simulink model "FOC_Simulate"  (R2016b)
settings: Solver=ode4  StartTime=0.0  StopTime=15  FixedStep=1e-5  RelTol=1e-3  EnableMultiTasking=on
undefined symbols (not defined in the file): sigbuilder_block
libraries: powerlib_meascontrol x4, powerlib x4, simulink x4
settings Model: ExtModeTrigDuration=8  Creator=tiend  LastModifiedBy=tiend

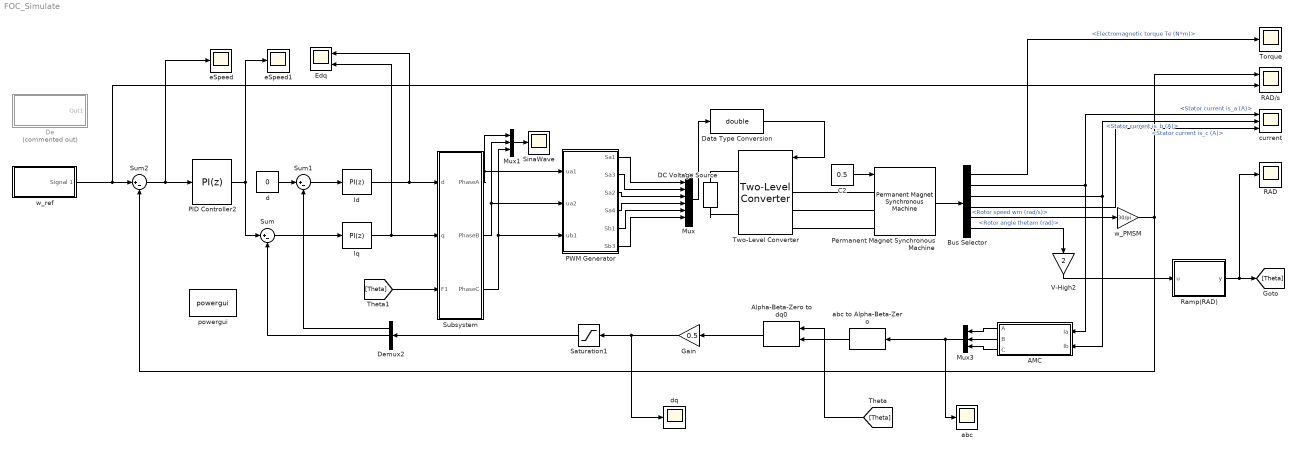
== system FOC_Simulate ==
  AMC : Subsystem
  Alpha-Beta-Zero to dq0 : powerlib_meascontrol/Transformations/Alpha-Beta-Zero to dq0  Alignment=Aligned with phase A axis
  Bus Selector : BusSelector  OutputSignals=Electromagnetic torque Te (N*m),Stator current is_a (A),Stator current is_b (A),Stator current is_c (A),Rotor speed wm (rad/s),Rotor angle thetam (rad)
  C2 : Constant  Value=0.5
  DC Voltage Source : powerlib/Electrical Sources/DC Voltage Source  Amplitude=300  Measurements=Voltage
  Data Type Conversion : DataTypeConversion  OutDataTypeStr=double
  De : Subsystem  Commented=on
  Demux2 : Demux  Outputs=3
  Edq : Scope  NumInputPorts=2
  Gain : Gain  Gain=0.5
  Id : simulink/Continuous/PID Controller  Controller=PI  TimeDomain=Discrete-time  SampleTime=-1  IntegratorMethod=Forward Euler  FilterMethod=Forward Euler  Form=Parallel  UseFilter=on  ControllerParametersSource=internal  P=5  I=0.3  D=0  N=100  InitialConditionSource=internal  InitialConditionForIntegrator=0  InitialConditionForFilter=0  ExternalReset=none  LimitOutput=on  UpperSaturationLimit=1  LowerSaturationLimit=-1  LinearizeAsGain=on  AntiWindupMode=none  Kb=1  TrackingMode=off  Kt=1  PParamMin=[]  PParamMax=[]  IParamMin=[]  IParamMax=[]  DParamMin=[]  DParamMax=[]  NParamMin=[]  NParamMax=[]  KbParamMin=[]  KbParamMax=[]  KtParamMin=[]  KtParamMax=[]  POutMin=[]  POutMax=[]  IOutMin=[]  IOutMax=[]  DOutMin=[]  DOutMax=[]  NOutMin=[]  NOutMax=[]  KbOutMin=[]  KbOutMax=[]  KtOutMin=[]  KtOutMax=[]  IntegratorOutMin=[]  IntegratorOutMax=[]  FilterOutMin=[]  FilterOutMax=[]  SumOutMin=[]  SumOutMax=[]  SumI1OutMin=[]  SumI1OutMax=[]  SumI2OutMin=[]  SumI2OutMax=[]  SumI3OutMin=[]  SumI3OutMax=[]  SumDOutMin=[]  SumDOutMax=[]  SaturationOutMin=[]  SaturationOutMax=[]  IntegratorContinuousStateAttributes=''  IntegratorStateMustResolveToSignalObject=off  IntegratorRTWStateStorageClass=Auto  FilterContinuousStateAttributes=''  FilterStateMustResolveToSignalObject=off  FilterRTWStateStorageClass=Auto  DifferentiatorICPrevScaledInput=0  DifferentiatorOutMin=[]  DifferentiatorOutMax=[]
  Iq : simulink/Continuous/PID Controller  Controller=PI  TimeDomain=Discrete-time  SampleTime=-1  IntegratorMethod=Forward Euler  FilterMethod=Forward Euler  Form=Parallel  UseFilter=on  ControllerParametersSource=internal  P=5  I=0.3  D=0  N=100  InitialConditionSource=internal  InitialConditionForIntegrator=0  InitialConditionForFilter=0  ExternalReset=none  LimitOutput=on  UpperSaturationLimit=1  LowerSaturationLimit=-1  LinearizeAsGain=on  AntiWindupMode=none  Kb=1  TrackingMode=off  Kt=1  PParamMin=[]  PParamMax=[]  IParamMin=[]  IParamMax=[]  DParamMin=[]  DParamMax=[]  NParamMin=[]  NParamMax=[]  KbParamMin=[]  KbParamMax=[]  KtParamMin=[]  KtParamMax=[]  POutMin=[]  POutMax=[]  IOutMin=[]  IOutMax=[]  DOutMin=[]  DOutMax=[]  NOutMin=[]  NOutMax=[]  KbOutMin=[]  KbOutMax=[]  KtOutMin=[]  KtOutMax=[]  IntegratorOutMin=[]  IntegratorOutMax=[]  FilterOutMin=[]  FilterOutMax=[]  SumOutMin=[]  SumOutMax=[]  SumI1OutMin=[]  SumI1OutMax=[]  SumI2OutMin=[]  SumI2OutMax=[]  SumI3OutMin=[]  SumI3OutMax=[]  SumDOutMin=[]  SumDOutMax=[]  SaturationOutMin=[]  SaturationOutMax=[]  IntegratorContinuousStateAttributes=''  IntegratorStateMustResolveToSignalObject=off  IntegratorRTWStateStorageClass=Auto  FilterContinuousStateAttributes=''  FilterStateMustResolveToSignalObject=off  FilterRTWStateStorageClass=Auto  DifferentiatorICPrevScaledInput=0  DifferentiatorOutMin=[]  DifferentiatorOutMax=[]
  Mux : Mux  Inputs=6
  Mux1 : Mux  Inputs=3
  Mux3 : Mux  Inputs=3
  PID Controller2 : simulink/Continuous/PID Controller  Controller=PI  TimeDomain=Discrete-time  SampleTime=-1  IntegratorMethod=Forward Euler  FilterMethod=Forward Euler  Form=Parallel  UseFilter=on  ControllerParametersSource=internal  P=1/900  I=0.005  D=0  N=100  InitialConditionSource=internal  InitialConditionForIntegrator=0  InitialConditionForFilter=0  ExternalReset=none  LimitOutput=off  UpperSaturationLimit=1  LowerSaturationLimit=-1  LinearizeAsGain=on  AntiWindupMode=none  Kb=1  TrackingMode=off  Kt=1  PParamMin=[]  PParamMax=[]  IParamMin=[]  IParamMax=[]  DParamMin=[]  DParamMax=[]  NParamMin=[]  NParamMax=[]  KbParamMin=[]  KbParamMax=[]  KtParamMin=[]  KtParamMax=[]  POutMin=[]  POutMax=[]  IOutMin=[]  IOutMax=[]  DOutMin=[]  DOutMax=[]  NOutMin=[]  NOutMax=[]  KbOutMin=[]  KbOutMax=[]  KtOutMin=[]  KtOutMax=[]  IntegratorOutMin=[]  IntegratorOutMax=[]  FilterOutMin=[]  FilterOutMax=[]  SumOutMin=[]  SumOutMax=[]  SumI1OutMin=[]  SumI1OutMax=[]  SumI2OutMin=[]  SumI2OutMax=[]  SumI3OutMin=[]  SumI3OutMax=[]  SumDOutMin=[]  SumDOutMax=[]  SaturationOutMin=[]  SaturationOutMax=[]  IntegratorContinuousStateAttributes=''  IntegratorStateMustResolveToSignalObject=off  IntegratorRTWStateStorageClass=Auto  FilterContinuousStateAttributes=''  FilterStateMustResolveToSignalObject=off  FilterRTWStateStorageClass=Auto  DifferentiatorICPrevScaledInput=0  DifferentiatorOutMin=[]  DifferentiatorOutMax=[]
  PWM Generator : Subsystem
  Permanent Magnet Synchronous Machine : powerlib/Machines/Permanent Magnet Synchronous Machine  NbPhases=3  FluxDistribution=Sinusoidal  RotorType=Round  MechanicalLoad=Torque Tm  PresetModel="01:  0.8 Nm 300 Vdc 3000 RPM - 0.8 Nm"  ShowDetailedParameters=on  MeasurementBus=off  Resistance=18.7  Inductance=8.5e-3  dqInductances=[0.02547 0.02816]  La=0.02682  MachineConstant=Flux linkage established by magnets (V.s)  Flux=0.1717  VoltageCst=62.2859  TorqueCst=0.5151  Flat=120  Mechanical=[2.26e-05 1.349e-05 2 0]  PolePairs=2  InitialConditions=[0,30, 0,0]  InitialConditions5ph=[0 0 0 0 0 0]  TsPowergui=0  TsBlock=-1  RefAngle=Aligned with phase A axis (original Park)
  RAD : Scope
  RAD/s : Scope  NumInputPorts=2
  Ramp(RAD) : MATLAB Function  TreatAsAtomicUnit=on
  Saturation1 : Saturate  UpperLimit=1  LowerLimit=-1
  SinaWave : Scope
  Subsystem : Subsystem
  Sum : Sum  Inputs=|+-
  Sum1 : Sum  Inputs=|+-
  Sum2 : Sum  Inputs=|+-
  Torque : Scope
  Two-Level Converter : powerlib/Power Electronics/Two-Level Converter  ModelType=Switching devices  Ron=1e-3  Rs=1e6  Cs=inf  Vforward=[0,0]  Ron_Diode=1e-3  Rs_Diode=1e6  Cs_Diode=inf  Vf_Diode=1e-3  Rs_CurrentSource=inf
  V-High2 : Gain  Gain=2
  abc : Scope
  abc to Alpha-Beta-Zero : powerlib_meascontrol/Transformations/abc to Alpha-Beta-Zero
  current : Scope  NumInputPorts=3
  d : Constant  Value=0
  dq : Scope
  eSpeed : Scope
  eSpeed1 : Scope
  powergui : powerlib/powergui  Priority=1  SimulationMode=Discrete  SolverType=Tustin/Backward Euler (TBE)  SampleTime=1e-5  frequency=60  SPID=off  DisableSnubberDevices=off  DisableRonSwitches=off  DisableVfSwitches=off  SwTol=0  DisplayEquations=off  Interpol=off  ExternalGateDelay=off  methode=off  Ts=10  FunctionMessages=off  echomessages=off  HookPort=off  EnableUseOfTLC=off  x0status=blocks  frequencyindice=0  Pbase=100e6  ErrMax=1e-4  Iterations=50  UnitsV=kV  UnitsW=MW  buscounter=0  RestoreLinks=warning  ResistiveCurrentMeasurement=off  Frange=[0:2:500]  Ylog=off  Xlog=on  ShowGrid=off  save=off  variable=ZData  structure=0  ZoomFFT=off  StartTime=0.0  cycles=1  DisplayStyle=1  fundamental=60  FreqAxis=off  MaxFrequency=1000  frequencyindicesteady=1  RmsSteady=1  display=off
  w_PMSM : Gain  Gain=30/pi
  w_ref : Subsystem  Tag=STV Subsys  LoadFcn=sigbuilder_block('load');  StartFcn=sigbuilder_block('start');  StopFcn=sigbuilder_block('stop');  ClipboardFcn=sigbuilder_block('clipboard');  mask(Sigbuilder block){tuvar=[0:10]}
      mask help: Simulink:masks:SigbuilderBlock_MD
      mask init:
      | if ~strcmp(get_param(bdroot(gcbh),'SimulationStatus'),'stopped') tuvar = sigbuilder_block('maskInit'); end
      settings: CopyFcn=sigbuilder_block('copy');  DeleteFcn=sigbuilder_block('delete');  ModelCloseFcn=sigbuilder_block('modelClose');  PreSaveFcn=sigbuilder_block('preSave');  PauseFcn=sigbuilder_block('pause');  ContinueFcn=sigbuilder_block('continue');  NameChangeFcn=sigbuilder_block('namechange');  OpenFcn=sigbuilder_block('open',[158.25 79.5 550.5 359.25 ]);  CloseFcn=sigbuilder_block('close');
      mask Display: plot(0, 0, 100, 100,[2, 2, 32, 32, 2], [68, 8, 8, 68, 68],[32, 2], [38, 38], [32, 19, 2],[53, 60, 44], [32, 17, 17, 2],[16, 16, 31, 31]);txt = getActiveGroup(gcbh);text(2, 100, txt,'verticalAlignment', 'top');
  wires:
  Subsystem/3(PhaseC) -> PWM Generator/3(ub1), Mux1/3
  Subsystem/2(PhaseB) -> PWM Generator/2(ua2), Mux1/2
  PWM Generator/3(Sa2) -> Mux/3
  PWM Generator/4(Sa4) -> Mux/4
  PWM Generator/2(Sa3) -> Mux/2
  PWM Generator/5(Sb1) -> Mux/5
  PWM Generator/1(Sa1) -> Mux/1
  PWM Generator/6(Sb3) -> Mux/6
  Mux/1 -> Data Type Conversion/1
  Data Type Conversion/1 -> Two-Level Converter/1
  Permanent Magnet Synchronous Machine/1 -> Bus Selector/1
  Mux1/1 -> SinaWave/1
  Subsystem/1(PhaseA) -> PWM Generator/1(ua1), Mux1/1
  Bus Selector/2 -> AMC/1(Ia), current/1  "<Stator current is_a (A)>"
  Bus Selector/3 -> AMC/2(Ib), current/2  "<Stator current is_b (A)>"
  Bus Selector/4 -> current/3  "<Stator current is_c (A)>"
  Bus Selector/6 -> V-High2/1  "<Rotor angle thetam (rad)>"
  AMC/3(C) -> Mux3/3
  AMC/2(B) -> Mux3/2
  AMC/1(A) -> Mux3/1
  Mux3/1 -> abc to Alpha-Beta-Zero/1, abc/1
  V-High2/1 -> Ramp(RAD)/1(u)
  Ramp(RAD)/1(y) -> RAD/1, [Theta]
  Bus Selector/5 -> w_PMSM/1  "<Rotor speed wm (rad/s)>"
  Gain/1 -> Saturation1/1, dq/1
  d/1 -> Sum1/1
  Sum1/1 -> Id/1
  Id/1 -> Subsystem/1(d), Edq/1
  Sum2/1 -> PID Controller2/1, eSpeed/1
  PID Controller2/1 -> Sum/1, eSpeed1/1
  Saturation1/1 -> Demux2/1
  Demux2/1 -> Sum1/2
  w_ref/1(Signal 1) -> RAD/s/2, Sum2/1
  Sum/1 -> Iq/1
  Demux2/2 -> Sum/2
  Iq/1 -> Subsystem/2(q), Edq/2
  abc to Alpha-Beta-Zero/1 -> Alpha-Beta-Zero to dq0/1
  Alpha-Beta-Zero to dq0/1 -> Gain/1
  w_PMSM/1 -> Sum2/2, RAD/s/1
  [Theta] -> Alpha-Beta-Zero to dq0/2
  [Theta] -> Subsystem/3(F1)
  Bus Selector/1 -> Torque/1  "<Electromagnetic torque Te (N*m)>"
  C2/1 -> Permanent Magnet Synchronous Machine/1
  connections:
  Two-Level Converter/LConn1 -- Permanent Magnet Synchronous Machine/LConn1
  Two-Level Converter/LConn2 -- Permanent Magnet Synchronous Machine/LConn2
  Two-Level Converter/LConn3 -- Permanent Magnet Synchronous Machine/LConn3
  DC Voltage Source/RConn1 -- Two-Level Converter/RConn1
  DC Voltage Source/LConn1 -- Two-Level Converter/RConn2

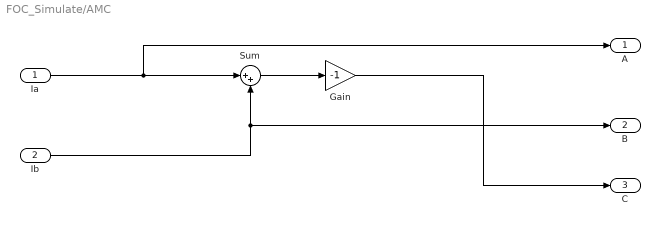
== system FOC_Simulate/AMC ==
  Ia : Inport
  Ib : Inport  Port=2
  Gain : Gain  Gain=-1
  Sum : Sum  Inputs=|++
  A : Outport
  B : Outport  Port=2
  C : Outport  Port=3
  wires:
  Sum/1 -> Gain/1
  Ia/1 -> A/1, Sum/1
  Ib/1 -> B/1, Sum/2
  Gain/1 -> C/1

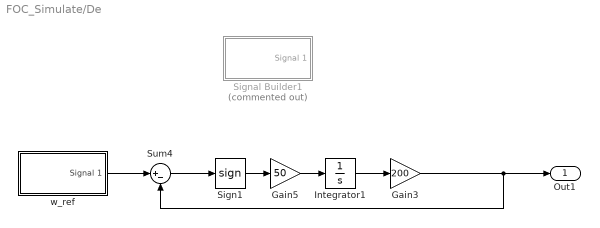
== system FOC_Simulate/De ==
  Gain3 : Gain  Gain=200
  Gain5 : Gain  Gain=50
  Integrator1 : Integrator
  Sign1 : Signum  ZeroCross=off
  Signal Builder1 : Subsystem  Tag=STV Subsys  Commented=on  LoadFcn=sigbuilder_block('load');  StartFcn=sigbuilder_block('start');  StopFcn=sigbuilder_block('stop');  ClipboardFcn=sigbuilder_block('clipboard');  mask(Sigbuilder block){tuvar=[0:10]}
      mask help: Simulink:masks:SigbuilderBlock_MD
      mask init:
      | if ~strcmp(get_param(bdroot(gcbh),'SimulationStatus'),'stopped') tuvar = sigbuilder_block('maskInit'); end
      settings: CopyFcn=sigbuilder_block('copy');  DeleteFcn=sigbuilder_block('delete');  ModelCloseFcn=sigbuilder_block('modelClose');  PreSaveFcn=sigbuilder_block('preSave');  PauseFcn=sigbuilder_block('pause');  ContinueFcn=sigbuilder_block('continue');  NameChangeFcn=sigbuilder_block('namechange');  OpenFcn=sigbuilder_block('open',[120 -80.25 550.5 359.25 ]);  CloseFcn=sigbuilder_block('close');
      mask Display: plot(0, 0, 100, 100,[2, 2, 32, 32, 2], [68, 8, 8, 68, 68],[32, 2], [38, 38], [32, 19, 2],[53, 60, 44], [32, 17, 17, 2],[16, 16, 31, 31]);txt = getActiveGroup(gcbh);text(2, 100, txt,'verticalAlignment', 'top');
  Sum4 : Sum  Inputs=|+-
  w_ref : Subsystem  Tag=STV Subsys  LoadFcn=sigbuilder_block('load');  StartFcn=sigbuilder_block('start');  StopFcn=sigbuilder_block('stop');  ClipboardFcn=sigbuilder_block('clipboard');  mask(Sigbuilder block){tuvar=[0:10]}
      mask help: Simulink:masks:SigbuilderBlock_MD
      mask init:
      | if ~strcmp(get_param(bdroot(gcbh),'SimulationStatus'),'stopped') tuvar = sigbuilder_block('maskInit'); end
      settings: CopyFcn=sigbuilder_block('copy');  DeleteFcn=sigbuilder_block('delete');  ModelCloseFcn=sigbuilder_block('modelClose');  PreSaveFcn=sigbuilder_block('preSave');  PauseFcn=sigbuilder_block('pause');  ContinueFcn=sigbuilder_block('continue');  NameChangeFcn=sigbuilder_block('namechange');  OpenFcn=sigbuilder_block('open',[158.25 79.5 550.5 359.25 ]);  CloseFcn=sigbuilder_block('close');
      mask Display: plot(0, 0, 100, 100,[2, 2, 32, 32, 2], [68, 8, 8, 68, 68],[32, 2], [38, 38], [32, 19, 2],[53, 60, 44], [32, 17, 17, 2],[16, 16, 31, 31]);txt = getActiveGroup(gcbh);text(2, 100, txt,'verticalAlignment', 'top');
  Out1 : Outport
  wires:
  w_ref/1(Signal 1) -> Sum4/1
  Integrator1/1 -> Gain3/1
  Sum4/1 -> Sign1/1
  Sign1/1 -> Gain5/1
  Gain5/1 -> Integrator1/1
  Gain3/1 -> Out1/1, Sum4/2

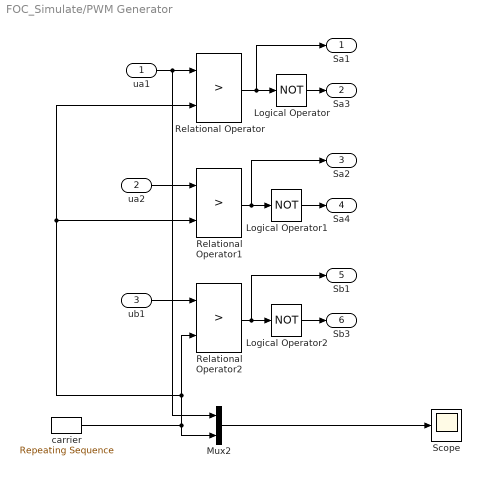
== system FOC_Simulate/PWM Generator ==
  ua1 : Inport
  ua2 : Inport  Port=2
  ub1 : Inport  Port=3
  Logical Operator : Logic  Operator=NOT  AllPortsSameDT=off  OutDataTypeStr=boolean
  Logical Operator1 : Logic  Operator=NOT  AllPortsSameDT=off  OutDataTypeStr=boolean
  Logical Operator2 : Logic  Operator=NOT  AllPortsSameDT=off  OutDataTypeStr=boolean
  Mux2 : Mux  Inputs=2
  Relational Operator : RelationalOperator  Operator=>  OutDataTypeStr=boolean  RndMeth=Nearest
  Relational Operator1 : RelationalOperator  Operator=>  OutDataTypeStr=boolean  RndMeth=Nearest
  Relational Operator2 : RelationalOperator  Operator=>  OutDataTypeStr=boolean  RndMeth=Nearest
  Scope : Scope
  carrier : simulink/Sources/Repeating Sequence  rep_seq_t=[0 1/20000 1/10000]  rep_seq_y=[0 1 0]
  Sa1 : Outport
  Sa3 : Outport  Port=2
  Sa2 : Outport  Port=3
  Sa4 : Outport  Port=4
  Sb1 : Outport  Port=5
  Sb3 : Outport  Port=6
  wires:
  Logical Operator2/1 -> Sb3/1
  Logical Operator1/1 -> Sa4/1
  ub1/1 -> Relational Operator2/1
  ua2/1 -> Relational Operator1/1
  Relational Operator2/1 -> Sb1/1, Logical Operator2/1
  Relational Operator1/1 -> Sa2/1, Logical Operator1/1
  ua1/1 -> Mux2/1, Relational Operator/1
  Relational Operator/1 -> Logical Operator/1, Sa1/1
  Logical Operator/1 -> Sa3/1
  carrier/1 -> Mux2/2, Relational Operator/2, Relational Operator1/2, Relational Operator2/2
  Mux2/1 -> Scope/1

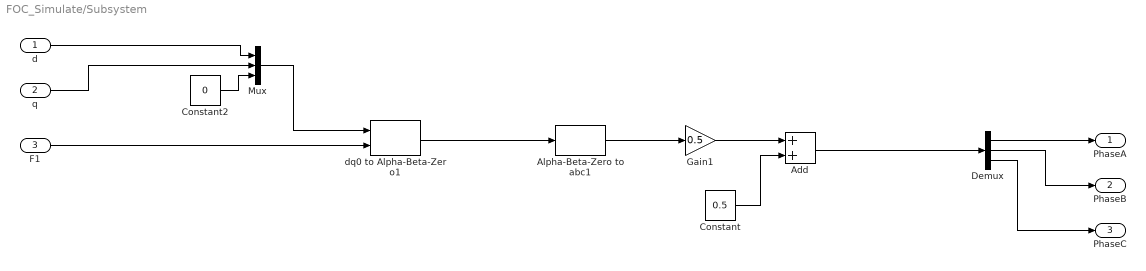
== system FOC_Simulate/Subsystem ==
  d : Inport
  q : Inport  Port=2
  F1 : Inport  Port=3
  Add : Sum
  Alpha-Beta-Zero to abc1 : powerlib_meascontrol/Transformations/Alpha-Beta-Zero to abc
  Constant : Constant  Value=0.5  SampleTime=-1
  Constant2 : Constant  Value=0  SampleTime=-1
  Demux : Demux  Outputs=3
  Gain1 : Gain  Gain=0.5
  Mux : Mux  Inputs=3
  dq0 to Alpha-Beta-Zero1 : powerlib_meascontrol/Transformations/dq0 to Alpha-Beta-Zero  Alignment=Aligned with phase A axis
  PhaseA : Outport
  PhaseB : Outport  Port=2
  PhaseC : Outport  Port=3
  wires:
  Constant/1 -> Add/2
  Alpha-Beta-Zero to abc1/1 -> Gain1/1
  Demux/1 -> PhaseA/1
  Demux/2 -> PhaseB/1
  Demux/3 -> PhaseC/1
  Mux/1 -> dq0 to Alpha-Beta-Zero1/1
  Add/1 -> Demux/1
  Constant2/1 -> Mux/3
  d/1 -> Mux/1
  Gain1/1 -> Add/1
  F1/1 -> dq0 to Alpha-Beta-Zero1/2
  q/1 -> Mux/2
  dq0 to Alpha-Beta-Zero1/1 -> Alpha-Beta-Zero to abc1/1

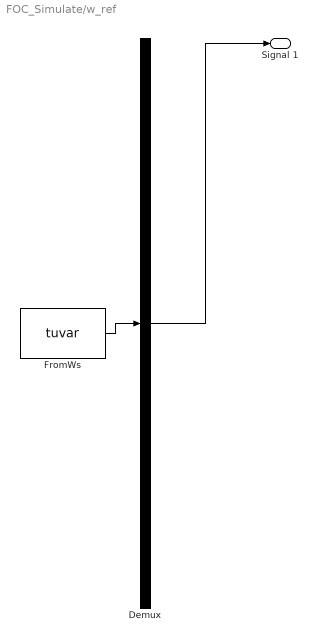
== system FOC_Simulate/w_ref ==
  Demux : Demux  Tag=STV Demux  Outputs=1
  FromWs : FromWorkspace  Tag=STV FromWs  VariableName=tuvar  SampleTime=0
      SigBuilderData=|
      | common.afterFinalStr = 'Extrapolate'
      | common.sampleTime = 0
      | dataSet.timeRange = [0 100]
      | dataSet.name = 'Group 1'
      | sbobj.Groups.Name = 'Group 1'
      | sbobj.Groups.Signals.Name = 'Signal 1'
      | sbobj.Groups.Signals.XData = [0 1 1 3.2 3.2 7 7 12 12 100]
      | sbobj.Groups.Signals.YData = [0 0 500 500 1500 1500 3000 3000 0 0]
      | sbobj.Groups.TimeRange = [0 100]
  Signal 1 : Outport  Tag=STV Outport
  wires:
  Demux/1 -> Signal 1/1
  FromWs/1 -> Demux/1

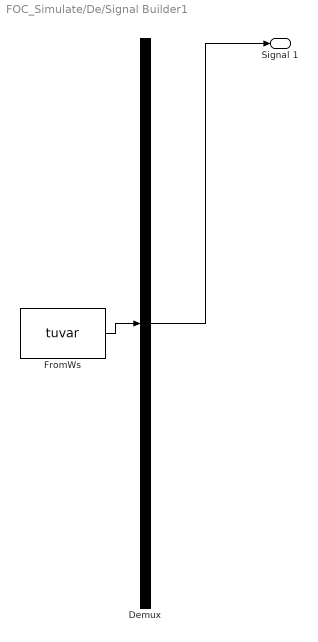
== system FOC_Simulate/De/Signal Builder1 ==
  Demux : Demux  Tag=STV Demux  Outputs=1
  FromWs : FromWorkspace  Tag=STV FromWs  VariableName=tuvar  SampleTime=0
      SigBuilderData=|
      | common.afterFinalStr = 'Extrapolate'
      | common.sampleTime = 0
      | dataSet.timeRange = [0 100]
      | dataSet.name = 'Group 1'
      | sbobj.Groups.Name = 'Group 1'
      | sbobj.Groups.Signals.Name = 'Signal 1'
      | sbobj.Groups.Signals.XData = [0 1 1 7 7 15 15 40 40 60 60 100]
      | sbobj.Groups.Signals.YData = [0 0 500 500 1500 1500 3000 3000 400 400 0 0]
      | sbobj.Groups.TimeRange = [0 100]
  Signal 1 : Outport  Tag=STV Outport
  wires:
  Demux/1 -> Signal 1/1
  FromWs/1 -> Demux/1

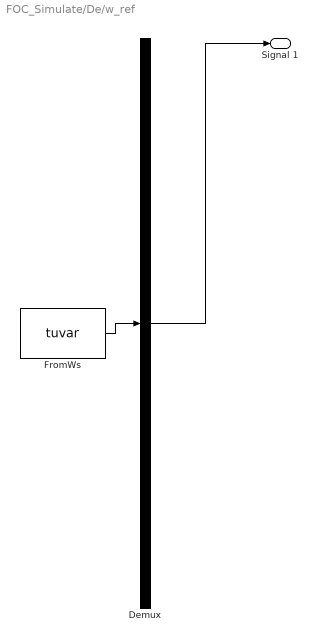
== system FOC_Simulate/De/w_ref ==
  Demux : Demux  Tag=STV Demux  Outputs=1
  FromWs : FromWorkspace  Tag=STV FromWs  VariableName=tuvar  SampleTime=0
      SigBuilderData=|
      | common.afterFinalStr = 'Extrapolate'
      | common.sampleTime = 0
      | dataSet.timeRange = [0 100]
      | dataSet.name = 'Group 1'
      | sbobj.Groups.Name = 'Group 1'
      | sbobj.Groups.Signals.Name = 'Signal 1'
      | sbobj.Groups.Signals.XData = [0 1 1 3.2 3.2 7 7 12 12 100]
      | sbobj.Groups.Signals.YData = [0 0 500 500 1500 1500 3000 3000 0 0]
      | sbobj.Groups.TimeRange = [0 100]
  Signal 1 : Outport  Tag=STV Outport
  wires:
  Demux/1 -> Signal 1/1
  FromWs/1 -> Demux/1

== matlab function FOC_Simulate/Ramp(RAD) ==
  data: u input; y output
function y = fcn(u)
if u>=(2*pi)
    u=mod(u,2*pi);
end
y = u;
